simulink model "ClosedLoop_System_Simulink"  (R2020a)
settings: Solver=ode4  StartTime=0.0  StopTime=t_final  FixedStep=dt  RelTol=1e-3
values from neighbouring files (symbols this model uses):
  e_IC = e_IC_1(i)    [HW3_c.m]    (also in HW3_e.m = 40.6)
  K = 60    [HW3_a.m]    (also in HW3_b.m = 100; HW3_c.m; HW3_d.m = 1; HW3_e.m = 100)
undefined symbols (not defined in the file or in its folder): A, B, C, D
settings Model: Creator=spect  LastModifiedBy=spect
settings DataIOCC: SaveFormat=Array  ReturnWorkspaceOutputs=off

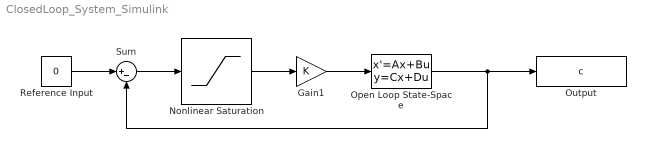
== system ClosedLoop_System_Simulink ==
  Gain1 : Gain  Gain=K
  Nonlinear Saturation : Saturate  UpperLimit=20  LowerLimit=-20
  Open Loop State-Space : StateSpace  A=A  B=B  C=C  D=D  InitialCondition=[0 0 -e_IC/500]
  Output : ToWorkspace  VariableName=c  SampleTime=-1
  Reference Input : Constant  Value=0
  Sum : Sum  Inputs=|+-
  wires:
  Reference Input/1 -> Sum/1
  Sum/1 -> Nonlinear Saturation/1
  Nonlinear Saturation/1 -> Gain1/1
  Gain1/1 -> Open Loop State-Space/1
  Open Loop State-Space/1 -> Output/1, Sum/2
